simulink model "Rider_Controls_OutHardware_CAN_Enable"  (R2014b)
settings: configuration reference "Embedded_Configuration" (kept outside this file)
PreLoadFcn:
  | load('Embedded_Config.mat')
PostLoadFcn:
  | c2000demoscallback(1)
model workspace: external: MAT-File Embedded_Config.mat (data not in the file)
undefined symbols (not defined in the file or in its folder): canChannel
libraries: canmsglib x2, canlib x2, realtime_pacer_lib x1, c280xlib x1
settings Model: Creator=The MathWorks Inc.  LastModifiedBy=Nathan

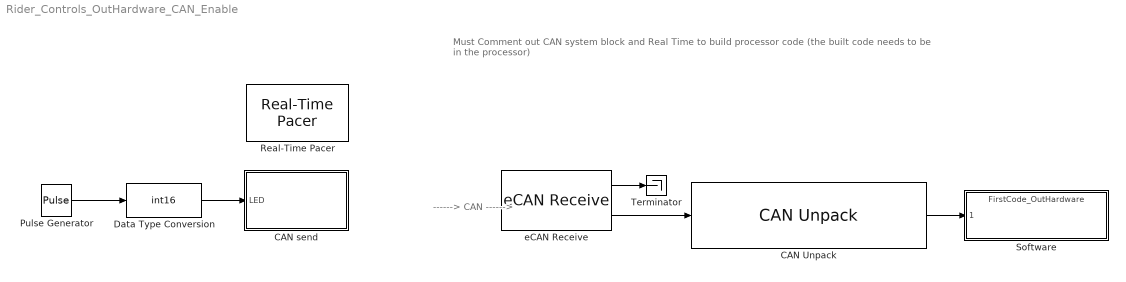
== system Rider_Controls_OutHardware_CAN_Enable ==
  note: Must Comment out CAN system block and Real Time
      | to build processor code
      | (the built code needs to be in the processor)
  note: ------> CAN ------>
  CAN Unpack : canmsglib/CAN Unpack  MsgList=(none)  MsgName=Button  MsgIDType=Standard (11-bit identifier)  MsgIdentifier=1  MsgLength=2  SignalInfo=LED$0$16$1$1$1$0$1$0$-Inf$Inf$#  NSignals=1  IDPort=off  TimestampPort=off  ErrorPort=off  RemotePort=off  LengthPort=off  StatusPort=off  StartBits=str2num('[int32(0)]')  SignalSizes=str2num('[int32(16)]')  ByteOrders=str2num('[int32(1)]')  DataTypes=str2num('[int32(1)]')  MultiplexTypes=str2num('[int32(1)]')  MultiplexValues=str2num('[double(0)]')  Factors=str2num('[double(1)]')  Offsets=str2num('[double(0)]')  Minimums=str2num('[double(-Inf)]')  Maximums=str2num('[double(Inf)]')
  CAN send : Subsystem
  Data Type Conversion : DataTypeConversion  OutDataTypeStr=int16  RndMeth=Nearest
  Pulse Generator : DiscretePulseGenerator  PulseType=Time based  Period=1  PulseWidth=50
  Real-Time Pacer : realtime_pacer_lib/Real-Time Pacer  simTimePerRealTime=1
  Software : ModelReference  ModelNameDialog=FirstCode_OutHardware.slx  SimulationMode=Normal  ModelReferenceVersion=1.87  CopyOfModelName=FirstCode_OutHardware.slx  DefaultDataLogging=on
  Terminator : Terminator
  eCAN Receive : c280xlib/eCAN Receive  chipFamily=C280x  useModule=eCAN_A  mailboxNo=0  messageID=1  messageType=Standard (11-bit identifier)  sampleTime=.01  dataType=CAN_MESSAGE_TYPE  initValue=0  outputMessageLength=off  outputMessageTimeStamp=off  postInterrupt=off  interruptLine=0
  wires:
  Pulse Generator/1 -> Data Type Conversion/1
  eCAN Receive/2 -> CAN Unpack/1
  eCAN Receive/1 -> Terminator/1
  CAN Unpack/1 -> Software/1
  Data Type Conversion/1 -> CAN send/1(LED)

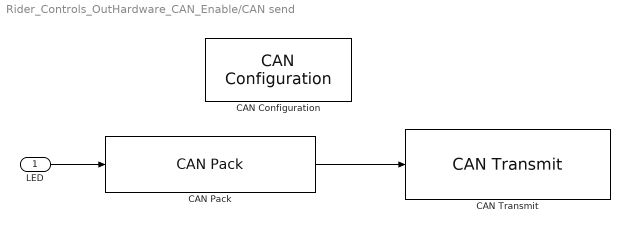
== system Rider_Controls_OutHardware_CAN_Enable/CAN send ==
  LED : Inport  OutDataTypeStr=int16
  CAN Configuration : canlib/CAN Configuration  BlockHandle=278.0035  DeviceMenu=Kvaser Eagle 1 (Channel 1)  Device=Kvaser Eagle 1 (Channel 1)  ObjConstructor=canChannel('Kvaser', 'Eagle 1', 1)  BusSpeed=500000  EnableBitParameters=off  SJW=1  TSEG1=4  TSEG2=3  NSamples=1  AckMode=Normal
  CAN Pack : canmsglib/CAN Pack  MsgList=(none)  MsgName=Button_Press  MsgIDType=Standard (11-bit identifier)  MsgIdentifier=1  MsgLength=2  SignalInfo=LED$0$16$1$1$1$0$1$0$-Inf$Inf$#  NSignals=1  StartBits=str2num('[int32(0)]')  SignalSizes=str2num('[int32(16)]')  ByteOrders=str2num('[int32(1)]')  DataTypes=str2num('[int32(1)]')  MultiplexTypes=str2num('[int32(1)]')  MultiplexValues=str2num('[double(0)]')  Factors=str2num('[double(1)]')  Offsets=str2num('[double(0)]')  Minimums=str2num('[double(-Inf)]')  Maximums=str2num('[double(Inf)]')  Remote=off
      settings: DataFormat=manually specified signals
  CAN Transmit : canlib/CAN Transmit  BlockHandle=284.0006  DeviceMenu=Kvaser Eagle 1 (Channel 1)  Device=Kvaser Eagle 1 (Channel 1)  ObjConstructor=canChannel('Kvaser', 'Eagle 1', 1)  EnablePeriodicTransmit=on  MessagePeriod=.01
  wires:
  LED/1 -> CAN Pack/1
  CAN Pack/1 -> CAN Transmit/1
